simulink model "NDT_Localization"  (R2022a)
settings: Solver=FixedStepAuto  StartTime=0.0  StopTime=10.0  RelTol=1e-3
model workspace (MAT data in the model file):
  SL_ROS_VariableLengthArrays_MaxSizes : object (value not decoded)
undefined symbols (not defined in the file or in its folder): null
libraries: ros2lib x9, robotlib x8, simulink x1
(part 5 of 12)

== system NDT_Localization/observation_callback/check_localizer/If Action Subsystem/register_measurement_impl/If Action Subsystem/If Action Subsystem/solve/If Action Subsystem1/For Iterator Subsystem/compute_next_step/If Action Subsystem1/psi_t ==
  a_t : Inport
  psi : Inport  Port=2
  localizer_ptr : Inport  Port=3
  Add : Sum  Inputs=+--
  Add1 : Sum  Inputs=+-
  Bus Creator : BusCreator  Inputs=3
  Bus Selector : BusSelector  OutputSignals=phi,mu
  Bus Selector1 : BusSelector  OutputSignals=value,derivative
  Bus Selector2 : BusSelector  OutputSignals=value,derivative
  Constant : Constant  Value=0.0
  If : If  NumInputs=2  IfExpression=u1 >= u2  ShowElse=off
  Product : Product  Inputs=3
  Product1 : Product
  initial_objective_function : Subsystem
  objective_function : Subsystem  TreatAsAtomicUnit=on
  psi_t : Outport
  wires:
  psi/1 -> Bus Selector/1
  a_t/1 -> Bus Creator/1, objective_function/1(step_size), Product/2, If/1  "a_t"
  If/1 -> objective_function/Action
  Constant/1 -> initial_objective_function/1(step_size), If/2
  Bus Selector/1 -> initial_objective_function/2(phi), objective_function/2(phi)  "<phi>"
  localizer_ptr/1 -> initial_objective_function/3(localizer_ptr), objective_function/3(localizer_ptr)
  Product/1 -> Add/3
  Bus Selector/2 -> Product1/1, Product/1  "<mu>"
  objective_function/1(objective_function_value) -> Bus Selector1/1
  Bus Selector1/1 -> Add/1  "<value>"
  initial_objective_function/1(initial_objective_function_value) -> Bus Selector2/1
  Bus Selector2/1 -> Add/2  "<value>"
  Bus Selector2/2 -> Product1/2, Product/3  "<derivative>"
  Add/1 -> Bus Creator/2  "value"
  Bus Selector1/2 -> Add1/1  "<derivative>"
  Product1/1 -> Add1/2
  Add1/1 -> Bus Creator/3  "derivative"
  Bus Creator/1 -> psi_t/1

== system NDT_Localization/observation_callback/check_localizer/If Action Subsystem/register_measurement_impl/If Action Subsystem/If Action Subsystem/solve/If Action Subsystem1/For Iterator Subsystem/compute_next_step/If Action Subsystem1/For Iterator Subsystem/If Action Subsystem ==
  localizer_ptr : Inport
  phi_t : Inport  Port=2
  psi_t : Inport  Port=3
  phi : Inport  Port=4
  psi : Inport  Port=5
  f_l : Inport  Port=6
  f_u : Inport  Port=7
  aux_function : Inport  Port=8
  Action Port : ActionPort  ActionPortLabel=if(u1 > 0)
  Bus Selector : BusSelector  OutputSignals=OptimizerT.MoreThuenteLineSearch.min_step
  Data Type Conversion : DataTypeConversion  SaturateOnIntegerOverflow=off  RndMeth=Floor
  Data Type Conversion1 : DataTypeConversion  OutDataTypeStr=uint8  SaturateOnIntegerOverflow=off  RndMeth=Floor
  If : If
  If Action Subsystem : Subsystem  TreatAsAtomicUnit=on
  If Action Subsystem1 : Subsystem  TreatAsAtomicUnit=on
  If Action Subsystem2 : Subsystem  TreatAsAtomicUnit=on
  If Action Subsystem3 : Subsystem  TreatAsAtomicUnit=on
  If1 : If
  Logical Operator : Logic  Operator=OR  AllPortsSameDT=off  OutDataTypeStr=boolean
  MATLAB Function : MATLAB Function  TreatAsAtomicUnit=on
  Merge : Merge
  Relational Operator : RelationalOperator  Operator=<  OutDataTypeStr=boolean  RndMeth=Simplest  InputSameDT=off
  Out1 : Outport
  aux_function_out : Outport  Port=2
  flag : Outport  Port=3
  wires:
  localizer_ptr/1 -> If Action Subsystem3/2(localizer_ptr), Bus Selector/1
  Bus Selector/1 -> Relational Operator/2  "<min_step>"
  aux_function/1 -> If Action Subsystem3/3(aux_function), Data Type Conversion/1
  Data Type Conversion/1 -> If/1
  If/1 -> If Action Subsystem/Action
  If/2 -> If Action Subsystem1/Action
  psi_t/1 -> If Action Subsystem/1(psi_t)
  phi_t/1 -> If Action Subsystem1/1(phi_t)
  f_l/1 -> If Action Subsystem/2(f_l), If Action Subsystem1/2(f_l)
  f_u/1 -> If Action Subsystem/3(f_u), If Action Subsystem1/3(f_u)
  If Action Subsystem/1(a_t) -> Merge/1
  If Action Subsystem1/1(a_t) -> Merge/2
  Merge/1 -> Relational Operator/1, If Action Subsystem3/1(a_t), MATLAB Function/1(a_t)
  MATLAB Function/1(y) -> Logical Operator/2
  Relational Operator/1 -> Logical Operator/1
  Logical Operator/1 -> Data Type Conversion1/1
  Data Type Conversion1/1 -> If1/1
  If1/1 -> If Action Subsystem2/Action
  If1/2 -> If Action Subsystem3/Action
  If Action Subsystem2/1(a_t_out) -> flag/1
  phi/1 -> If Action Subsystem3/4(phi)
  psi/1 -> If Action Subsystem3/5(psi)

== system NDT_Localization/observation_callback/check_localizer/If Action Subsystem/register_measurement_impl/If Action Subsystem/If Action Subsystem/solve/If Action Subsystem1/For Iterator Subsystem/compute_next_step/If Action Subsystem1/f_l/initial_objective_function ==
  step_size : Inport
  phi : Inport  Port=2
  localizer_ptr : Inport  Port=3
  Add : Sum
  Add4 : Sum  Inputs=+
  Bus Creator : BusCreator  Inputs=3
  Bus Selector : BusSelector  OutputSignals=eig_pose,opt_direction,problem
  Bus Selector1 : BusSelector  OutputSignals=scan,map
  Bus Selector2 : BusSelector  OutputSignals=vx.centroid,vx.inv_covariance
  Bus Selector3 : BusSelector  OutputSignals=outlier_ratio,localizer_config.map_config.voxel_size.x,localizer_config.map_config.voxel_size.y,localizer_config.map_config.voxel_size.z
  For Iterator Subsystem : Subsystem  TreatAsAtomicUnit=on
  Math Function2 : Math  Operator=square
  Product : Product
  Product{1..9} (9 alike) : Product  Multiplication=Matrix(*)
  angle_params : Subsystem
  gradient_angle : Subsystem
  point_gradient : MATLAB Function  TreatAsAtomicUnit=on
  set_jacobian : MATLAB Function  TreatAsAtomicUnit=on
  initial_objective_function_value : Outport
  wires:
  angle_params/1(params) -> gradient_angle/1(params)
  Bus Selector3/1 -> For Iterator Subsystem/4(outlier_ratio)  "<outlier_ratio>"
  gradient_angle/3(ga_c_out) -> Product4/2
  gradient_angle/4(ga_d_out) -> Product5/2
  gradient_angle/1(ga_a_out) -> Product2/2
  gradient_angle/6(ga_f_out) -> Product7/2
  Bus Selector2/2 -> For Iterator Subsystem/3(sigma)  "<inv_covariance>"
  Product5/1 -> point_gradient/4(ga_d)
  Product3/1 -> point_gradient/2(ga_b)
  set_jacobian/1(jacobian) -> For Iterator Subsystem/8(set_jacobian)
  Bus Selector1/1 -> Product9/1, Product8/1, Product7/1, Product6/1, Product5/1, Product4/1, Product3/1, Product2/1, For Iterator Subsystem/1(data)  "<scan>"
  Bus Selector/1 -> Add/1  "<eig_pose>"
  gradient_angle/7(ga_g_out) -> Product8/2
  Product8/1 -> point_gradient/7(ga_g)
  gradient_angle/8(ga_h_out) -> Product9/2
  Math Function2/1 -> Add4/1
  Product6/1 -> point_gradient/5(ga_e)
  Bus Selector2/1 -> For Iterator Subsystem/2(myu)  "<centroid>"
  localizer_ptr/1 -> Bus Selector3/1
  gradient_angle/5(ga_e_out) -> Product6/2
  gradient_angle/2(ga_b_out) -> Product3/2
  Add/1 -> Product/1
  Bus Selector/3 -> Bus Selector1/1  "<problem>"
  Product7/1 -> point_gradient/6(ga_f)
  Product9/1 -> point_gradient/8(ga_h)
  For Iterator Subsystem/2(jacobian_out) -> Product1/1
  Product/1 -> angle_params/1(pose)  "current_state"
  Add4/1 -> Product1/2, Product/2  "step_direction"
  Product2/1 -> point_gradient/1(ga_a)
  Bus Selector/2 -> Math Function2/1  "<opt_direction>"
  Bus Creator/1 -> initial_objective_function_value/1
  Bus Selector1/2 -> Bus Selector2/1  "<map>"
  point_gradient/1(hessian) -> For Iterator Subsystem/9(set_gradient)
  Bus Selector3/3 -> For Iterator Subsystem/6(voxel_size_y)  "<y>"
  Bus Selector3/4 -> For Iterator Subsystem/7(voxel_size_z)  "<z>"
  phi/1 -> Bus Selector/1
  Bus Selector3/2 -> For Iterator Subsystem/5(voxel_size_x)  "<x>"
  Product4/1 -> point_gradient/3(ga_c)
  step_size/1 -> Bus Creator/1, Add/2  "step_size"
  For Iterator Subsystem/1(score_out) -> Bus Creator/2  "value"
  Product1/1 -> Bus Creator/3  "derivative"

== system NDT_Localization/observation_callback/check_localizer/If Action Subsystem/register_measurement_impl/If Action Subsystem/If Action Subsystem/solve/If Action Subsystem1/For Iterator Subsystem/compute_next_step/If Action Subsystem1/f_l/objective_function ==
  step_size : Inport
  phi : Inport  Port=2
  localizer_ptr : Inport  Port=3
  Action Port : ActionPort
  Add : Sum
  Add4 : Sum  Inputs=+
  Bus Creator : BusCreator  Inputs=3
  Bus Selector : BusSelector  OutputSignals=eig_pose,opt_direction,problem
  Bus Selector1 : BusSelector  OutputSignals=scan,map
  Bus Selector2 : BusSelector  OutputSignals=vx.centroid,vx.inv_covariance
  Bus Selector3 : BusSelector  OutputSignals=outlier_ratio,localizer_config.map_config.voxel_size.x,localizer_config.map_config.voxel_size.y,localizer_config.map_config.voxel_size.z
  For Iterator Subsystem : Subsystem  TreatAsAtomicUnit=on
  Math Function2 : Math  Operator=square
  Product : Product
  Product{1..9} (9 alike) : Product  Multiplication=Matrix(*)
  angle_params : Subsystem
  gradient_angle : Subsystem
  point_gradient : MATLAB Function  TreatAsAtomicUnit=on
  set_jacobian : MATLAB Function  TreatAsAtomicUnit=on
  objective_function_value : Outport
  wires:
  Add/1 -> Product/1
  step_size/1 -> Bus Creator/1, Add/2  "step_size"
  Product/1 -> angle_params/1(pose)  "current_state"
  Bus Selector/1 -> Add/1  "<eig_pose>"
  Add4/1 -> Product1/2, Product/2  "step_direction"
  phi/1 -> Bus Selector/1
  Bus Selector/2 -> Math Function2/1  "<opt_direction>"
  Math Function2/1 -> Add4/1
  Bus Selector/3 -> Bus Selector1/1  "<problem>"
  For Iterator Subsystem/2(jacobian_out) -> Product1/1
  Product1/1 -> Bus Creator/3  "derivative"
  Product9/1 -> point_gradient/8(ga_h)
  Product8/1 -> point_gradient/7(ga_g)
  Bus Selector2/2 -> For Iterator Subsystem/3(sigma)  "<inv_covariance>"
  gradient_angle/4(ga_d_out) -> Product5/2
  Product7/1 -> point_gradient/6(ga_f)
  Product6/1 -> point_gradient/5(ga_e)
  gradient_angle/6(ga_f_out) -> Product7/2
  Bus Selector1/1 -> Product9/1, Product8/1, Product7/1, Product6/1, Product5/1, Product4/1, Product3/1, Product2/1, For Iterator Subsystem/1(data)  "<scan>"
  point_gradient/1(hessian) -> For Iterator Subsystem/9(set_gradient)
  gradient_angle/2(ga_b_out) -> Product3/2
  gradient_angle/3(ga_c_out) -> Product4/2
  gradient_angle/7(ga_g_out) -> Product8/2
  gradient_angle/5(ga_e_out) -> Product6/2
  gradient_angle/8(ga_h_out) -> Product9/2
  Product5/1 -> point_gradient/4(ga_d)
  Product3/1 -> point_gradient/2(ga_b)
  Product4/1 -> point_gradient/3(ga_c)
  angle_params/1(params) -> gradient_angle/1(params)
  set_jacobian/1(jacobian) -> For Iterator Subsystem/8(set_jacobian)
  Bus Selector1/2 -> Bus Selector2/1  "<map>"
  gradient_angle/1(ga_a_out) -> Product2/2
  Product2/1 -> point_gradient/1(ga_a)
  Bus Selector2/1 -> For Iterator Subsystem/2(myu)  "<centroid>"
  localizer_ptr/1 -> Bus Selector3/1
  Bus Selector3/1 -> For Iterator Subsystem/4(outlier_ratio)  "<outlier_ratio>"
  Bus Selector3/2 -> For Iterator Subsystem/5(voxel_size_x)  "<x>"
  Bus Selector3/3 -> For Iterator Subsystem/6(voxel_size_y)  "<y>"
  Bus Selector3/4 -> For Iterator Subsystem/7(voxel_size_z)  "<z>"
  For Iterator Subsystem/1(score_out) -> Bus Creator/2  "value"
  Bus Creator/1 -> objective_function_value/1

== system NDT_Localization/observation_callback/check_localizer/If Action Subsystem/register_measurement_impl/If Action Subsystem/If Action Subsystem/solve/If Action Subsystem1/For Iterator Subsystem/compute_next_step/If Action Subsystem1/f_u/initial_objective_function ==
  step_size : Inport
  phi : Inport  Port=2
  localizer_ptr : Inport  Port=3
  Add : Sum
  Add4 : Sum  Inputs=+
  Bus Creator : BusCreator  Inputs=3
  Bus Selector : BusSelector  OutputSignals=eig_pose,opt_direction,problem
  Bus Selector1 : BusSelector  OutputSignals=scan,map
  Bus Selector2 : BusSelector  OutputSignals=vx.centroid,vx.inv_covariance
  Bus Selector3 : BusSelector  OutputSignals=outlier_ratio,localizer_config.map_config.voxel_size.x,localizer_config.map_config.voxel_size.y,localizer_config.map_config.voxel_size.z
  For Iterator Subsystem : Subsystem  TreatAsAtomicUnit=on
  Math Function2 : Math  Operator=square
  Product : Product
  Product{1..9} (9 alike) : Product  Multiplication=Matrix(*)
  angle_params : Subsystem
  gradient_angle : Subsystem
  point_gradient : MATLAB Function  TreatAsAtomicUnit=on
  set_jacobian : MATLAB Function  TreatAsAtomicUnit=on
  initial_objective_function_value : Outport
  wires:
  angle_params/1(params) -> gradient_angle/1(params)
  Bus Selector3/1 -> For Iterator Subsystem/4(outlier_ratio)  "<outlier_ratio>"
  gradient_angle/3(ga_c_out) -> Product4/2
  gradient_angle/4(ga_d_out) -> Product5/2
  gradient_angle/1(ga_a_out) -> Product2/2
  gradient_angle/6(ga_f_out) -> Product7/2
  Bus Selector2/2 -> For Iterator Subsystem/3(sigma)  "<inv_covariance>"
  Product5/1 -> point_gradient/4(ga_d)
  Product3/1 -> point_gradient/2(ga_b)
  set_jacobian/1(jacobian) -> For Iterator Subsystem/8(set_jacobian)
  Bus Selector1/1 -> Product9/1, Product8/1, Product7/1, Product6/1, Product5/1, Product4/1, Product3/1, Product2/1, For Iterator Subsystem/1(data)  "<scan>"
  Bus Selector/1 -> Add/1  "<eig_pose>"
  gradient_angle/7(ga_g_out) -> Product8/2
  Product8/1 -> point_gradient/7(ga_g)
  gradient_angle/8(ga_h_out) -> Product9/2
  Math Function2/1 -> Add4/1
  Product6/1 -> point_gradient/5(ga_e)
  Bus Selector2/1 -> For Iterator Subsystem/2(myu)  "<centroid>"
  localizer_ptr/1 -> Bus Selector3/1
  gradient_angle/5(ga_e_out) -> Product6/2
  gradient_angle/2(ga_b_out) -> Product3/2
  Add/1 -> Product/1
  Bus Selector/3 -> Bus Selector1/1  "<problem>"
  Product7/1 -> point_gradient/6(ga_f)
  Product9/1 -> point_gradient/8(ga_h)
  For Iterator Subsystem/2(jacobian_out) -> Product1/1
  Product/1 -> angle_params/1(pose)  "current_state"
  Add4/1 -> Product1/2, Product/2  "step_direction"
  Product2/1 -> point_gradient/1(ga_a)
  Bus Selector/2 -> Math Function2/1  "<opt_direction>"
  Bus Creator/1 -> initial_objective_function_value/1
  Bus Selector1/2 -> Bus Selector2/1  "<map>"
  point_gradient/1(hessian) -> For Iterator Subsystem/9(set_gradient)
  Bus Selector3/3 -> For Iterator Subsystem/6(voxel_size_y)  "<y>"
  Bus Selector3/4 -> For Iterator Subsystem/7(voxel_size_z)  "<z>"
  phi/1 -> Bus Selector/1
  Bus Selector3/2 -> For Iterator Subsystem/5(voxel_size_x)  "<x>"
  Product4/1 -> point_gradient/3(ga_c)
  step_size/1 -> Bus Creator/1, Add/2  "step_size"
  For Iterator Subsystem/1(score_out) -> Bus Creator/2  "value"
  Product1/1 -> Bus Creator/3  "derivative"

== system NDT_Localization/observation_callback/check_localizer/If Action Subsystem/register_measurement_impl/If Action Subsystem/If Action Subsystem/solve/If Action Subsystem1/For Iterator Subsystem/compute_next_step/If Action Subsystem1/f_u/objective_function ==
  step_size : Inport
  phi : Inport  Port=2
  localizer_ptr : Inport  Port=3
  Action Port : ActionPort
  Add : Sum
  Add4 : Sum  Inputs=+
  Bus Creator : BusCreator  Inputs=3
  Bus Selector : BusSelector  OutputSignals=eig_pose,opt_direction,problem
  Bus Selector1 : BusSelector  OutputSignals=scan,map
  Bus Selector2 : BusSelector  OutputSignals=vx.centroid,vx.inv_covariance
  Bus Selector3 : BusSelector  OutputSignals=outlier_ratio,localizer_config.map_config.voxel_size.x,localizer_config.map_config.voxel_size.y,localizer_config.map_config.voxel_size.z
  For Iterator Subsystem : Subsystem  TreatAsAtomicUnit=on
  Math Function2 : Math  Operator=square
  Product : Product
  Product{1..9} (9 alike) : Product  Multiplication=Matrix(*)
  angle_params : Subsystem
  gradient_angle : Subsystem
  point_gradient : MATLAB Function  TreatAsAtomicUnit=on
  set_jacobian : MATLAB Function  TreatAsAtomicUnit=on
  objective_function_value : Outport
  wires:
  Add/1 -> Product/1
  step_size/1 -> Bus Creator/1, Add/2  "step_size"
  Product/1 -> angle_params/1(pose)  "current_state"
  Bus Selector/1 -> Add/1  "<eig_pose>"
  Add4/1 -> Product1/2, Product/2  "step_direction"
  phi/1 -> Bus Selector/1
  Bus Selector/2 -> Math Function2/1  "<opt_direction>"
  Math Function2/1 -> Add4/1
  Bus Selector/3 -> Bus Selector1/1  "<problem>"
  For Iterator Subsystem/2(jacobian_out) -> Product1/1
  Product1/1 -> Bus Creator/3  "derivative"
  Product9/1 -> point_gradient/8(ga_h)
  Product8/1 -> point_gradient/7(ga_g)
  Bus Selector2/2 -> For Iterator Subsystem/3(sigma)  "<inv_covariance>"
  gradient_angle/4(ga_d_out) -> Product5/2
  Product7/1 -> point_gradient/6(ga_f)
  Product6/1 -> point_gradient/5(ga_e)
  gradient_angle/6(ga_f_out) -> Product7/2
  Bus Selector1/1 -> Product9/1, Product8/1, Product7/1, Product6/1, Product5/1, Product4/1, Product3/1, Product2/1, For Iterator Subsystem/1(data)  "<scan>"
  point_gradient/1(hessian) -> For Iterator Subsystem/9(set_gradient)
  gradient_angle/2(ga_b_out) -> Product3/2
  gradient_angle/3(ga_c_out) -> Product4/2
  gradient_angle/7(ga_g_out) -> Product8/2
  gradient_angle/5(ga_e_out) -> Product6/2
  gradient_angle/8(ga_h_out) -> Product9/2
  Product5/1 -> point_gradient/4(ga_d)
  Product3/1 -> point_gradient/2(ga_b)
  Product4/1 -> point_gradient/3(ga_c)
  angle_params/1(params) -> gradient_angle/1(params)
  set_jacobian/1(jacobian) -> For Iterator Subsystem/8(set_jacobian)
  Bus Selector1/2 -> Bus Selector2/1  "<map>"
  gradient_angle/1(ga_a_out) -> Product2/2
  Product2/1 -> point_gradient/1(ga_a)
  Bus Selector2/1 -> For Iterator Subsystem/2(myu)  "<centroid>"
  localizer_ptr/1 -> Bus Selector3/1
  Bus Selector3/1 -> For Iterator Subsystem/4(outlier_ratio)  "<outlier_ratio>"
  Bus Selector3/2 -> For Iterator Subsystem/5(voxel_size_x)  "<x>"
  Bus Selector3/3 -> For Iterator Subsystem/6(voxel_size_y)  "<y>"
  Bus Selector3/4 -> For Iterator Subsystem/7(voxel_size_z)  "<z>"
  For Iterator Subsystem/1(score_out) -> Bus Creator/2  "value"
  Bus Creator/1 -> objective_function_value/1

== system NDT_Localization/observation_callback/check_localizer/If Action Subsystem/register_measurement_impl/If Action Subsystem/If Action Subsystem/solve/If Action Subsystem1/For Iterator Subsystem/compute_next_step/If Action Subsystem1/phi_0/For Iterator Subsystem ==
  data : Inport
  myu : Inport  Port=2
  sigma : Inport  Port=3
  outlier_ratio : Inport  Port=4
  voxel_size_x : Inport  Port=5
  voxel_size_y : Inport  Port=6
  voxel_size_z : Inport  Port=7
  set_jacobian : Inport  Port=8
  set_gradient : Inport  Port=9
  Affine : MATLAB Function  TreatAsAtomicUnit=on
  Delay : Delay  DelayLength=1
  For Iterator : ForIterator  IterationSource=external
  MATLAB Function : MATLAB Function  TreatAsAtomicUnit=on
  Width : Width
  gradient_jaco : Subsystem
  make_c_param : Subsystem
  make_d_param : Subsystem
  score : Subsystem
  score_out : Outport
  jacobian_out : Outport  Port=2
  wires:
  make_c_param/1(c1) -> make_d_param/1(c1)
  voxel_size_z/1 -> make_c_param/4(voxel_size_z)
  outlier_ratio/1 -> make_c_param/1(outlier_ratio)
  make_d_param/2(d2) -> gradient_jaco/9(d2), score/6(d2)
  voxel_size_y/1 -> make_c_param/3(voxel_size_y)
  make_c_param/2(c2) -> make_d_param/2(c2)
  voxel_size_x/1 -> make_c_param/2(voxel_size_x)
  make_d_param/1(d1) -> score/5(d1), gradient_jaco/8(d1)
  Width/1 -> For Iterator/1
  For Iterator/1 -> gradient_jaco/3(index), MATLAB Function/2(index)
  MATLAB Function/1(pt) -> Affine/1(u)
  Affine/1(out) -> score/4(x), gradient_jaco/4(data)
  sigma/1 -> score/2(sigma), gradient_jaco/5(sigma)
  myu/1 -> gradient_jaco/6(myu), score/3(myu)
  score/1(p) -> score_out/1, Delay/1
  Delay/1 -> score/1(score)
  set_jacobian/1 -> gradient_jaco/1(set_jacobian)
  gradient_jaco/1(Out1) -> jacobian_out/1
  set_gradient/1 -> gradient_jaco/2(set_gradient)
  data/1 -> gradient_jaco/7(x), MATLAB Function/1(data), Width/1

== system NDT_Localization/observation_callback/check_localizer/If Action Subsystem/register_measurement_impl/If Action Subsystem/If Action Subsystem/solve/If Action Subsystem1/For Iterator Subsystem/compute_next_step/If Action Subsystem1/phi_0/angle_params ==
  pose : Inport
  Bus Creator : BusCreator  Inputs=6
  If : If  NumInputs=2  IfExpression=u1 > u2
  If Action Subsystem : Subsystem  TreatAsAtomicUnit=on
  If Action Subsystem1 : Subsystem  TreatAsAtomicUnit=on
  If Action Subsystem2 : Subsystem  TreatAsAtomicUnit=on
  If Action Subsystem3 : Subsystem  TreatAsAtomicUnit=on
  If Action Subsystem4 : Subsystem  TreatAsAtomicUnit=on
  If Action Subsystem5 : Subsystem  TreatAsAtomicUnit=on
  If1 : If  NumInputs=2  IfExpression=u1 > u2
  If2 : If  NumInputs=2  IfExpression=u1 > u2
  MATLAB Function : MATLAB Function  TreatAsAtomicUnit=on
  Merge{,1..5} (6 alike) : Merge
  approx_thresh : Constant  Value=0.00010
  params : Outport
  wires:
  pose/1 -> MATLAB Function/1(u)
  MATLAB Function/1(x) -> If/2, If Action Subsystem1/1(x)
  MATLAB Function/3(z) -> If2/2, If Action Subsystem5/1(z)
  MATLAB Function/2(y) -> If Action Subsystem3/1(y), If1/2
  If Action Subsystem1/1(Out1) -> Merge/2
  If Action Subsystem1/2(Out2) -> Merge1/2
  If Action Subsystem3/1(Out1) -> Merge2/2
  If Action Subsystem3/2(Out2) -> Merge3/2
  If Action Subsystem5/1(Out1) -> Merge4/2
  If Action Subsystem5/2(Out2) -> Merge5/2
  approx_thresh/1 -> If2/1, If1/1, If/1
  If/1 -> If Action Subsystem/Action
  If/2 -> If Action Subsystem1/Action
  If1/1 -> If Action Subsystem2/Action
  If1/2 -> If Action Subsystem3/Action
  If2/2 -> If Action Subsystem5/Action
  If2/1 -> If Action Subsystem4/Action
  If Action Subsystem/1(Out1) -> Merge/1
  If Action Subsystem/2(Out2) -> Merge1/1
  If Action Subsystem2/1(Out1) -> Merge2/1
  If Action Subsystem2/2(Out2) -> Merge3/1
  If Action Subsystem4/1(Out1) -> Merge4/1
  If Action Subsystem4/2(Out2) -> Merge5/1
  Bus Creator/1 -> params/1
  Merge/1 -> Bus Creator/1  "cx"
  Merge1/1 -> Bus Creator/2  "sx"
  Merge2/1 -> Bus Creator/3  "cy"
  Merge3/1 -> Bus Creator/4  "sy"
  Merge4/1 -> Bus Creator/5  "cz"
  Merge5/1 -> Bus Creator/6  "sz"

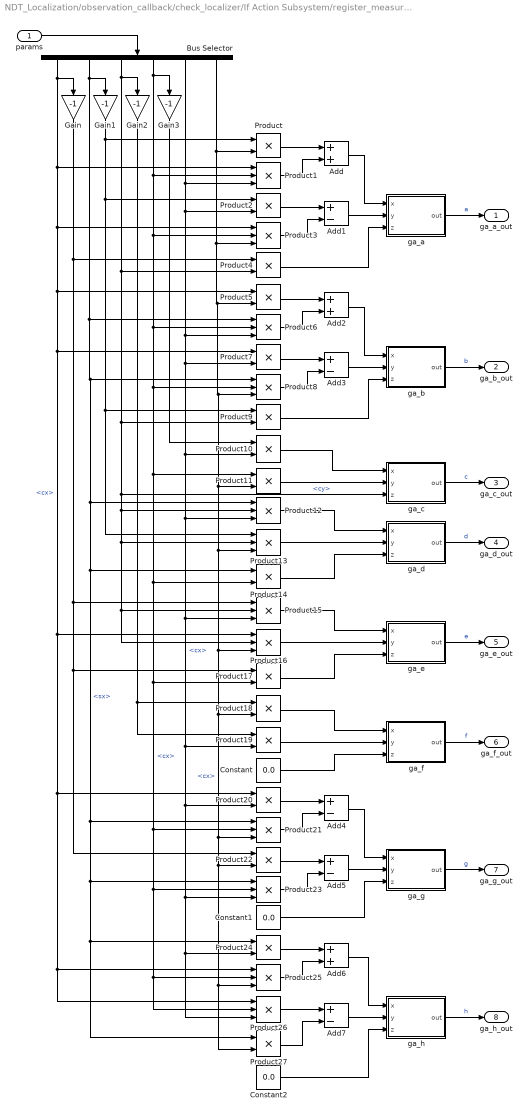
== system NDT_Localization/observation_callback/check_localizer/If Action Subsystem/register_measurement_impl/If Action Subsystem/If Action Subsystem/solve/If Action Subsystem1/For Iterator Subsystem/compute_next_step/If Action Subsystem1/phi_0/gradient_angle ==
  params : Inport
  Add : Sum
  Add{1,3..5,7} (5 alike) : Sum  Inputs=+-
  Add2 : Sum
  Add6 : Sum
  Bus Selector : BusSelector  OutputSignals=cx,sx,cy,sy,cz,sz
  Constant : Constant  Value=0.0
  Constant1 : Constant  Value=0.0
  Constant2 : Constant  Value=0.0
  Gain{,1..3} (4 alike) : Gain  Gain=-1
  Product{,2,4..5,7,9..11,14,17..20,22,24,27} (16 alike) : Product
  Product{1,3,6,8,12..13,15..16,21,23,25..26} (12 alike) : Product  Inputs=3
  ga_a : MATLAB Function  TreatAsAtomicUnit=on
  ga_b : MATLAB Function  TreatAsAtomicUnit=on
  ga_c : MATLAB Function  TreatAsAtomicUnit=on
  ga_d : MATLAB Function  TreatAsAtomicUnit=on
  ga_e : MATLAB Function  TreatAsAtomicUnit=on
  ga_f : MATLAB Function  TreatAsAtomicUnit=on
  ga_g : MATLAB Function  TreatAsAtomicUnit=on
  ga_h : MATLAB Function  TreatAsAtomicUnit=on
  ga_a_out : Outport
  ga_b_out : Outport  Port=2
  ga_c_out : Outport  Port=3
  ga_d_out : Outport  Port=4
  ga_e_out : Outport  Port=5
  ga_f_out : Outport  Port=6
  ga_g_out : Outport  Port=7
  ga_h_out : Outport  Port=8
  wires:
  params/1 -> Bus Selector/1
  Bus Selector/1 -> Product1/1, Product16/1, Product25/1, Product26/1, Product20/1, Product7/1, Product5/1, Product3/1, Gain/1  "<cx>"
  Bus Selector/2 -> Product6/1, Product12/1, Product14/1, Product21/1, Product23/1, Product27/1, Product24/1, Product8/1, Gain1/1  "<sx>"
  Bus Selector/3 -> Product12/2, Product13/2, Product15/2, Product16/2, ga_c/3(z), Product9/2, Product4/2, Gain2/1  "<cy>"
  Bus Selector/4 -> Product11/1, Product14/2, Product17/2, Product21/2, Product25/2, Product26/2, Product23/2, Product8/2, Product6/2, Product3/2, Product1/2, Gain3/1  "<cx>"
  Bus Selector/5 -> Product6/3, Product10/2, Product12/3, Product15/3, Product19/2, Product20/2, Product23/3, Product26/3, Product24/2, Product7/2, Product2/2, Product1/3  "<cx>"
  Bus Selector/6 -> Product11/2, Product13/3, Product16/3, Product18/2, Product21/3, Product22/2, Product25/3, Product27/2, Product8/3, Product5/2, Product3/3, Product/2  "<cx>"
  Gain1/1 -> Product13/1, Product9/1, Product2/1, Product/1
  Product/1 -> Add/1
  Product1/1 -> Add/2
  Product2/1 -> Add1/1
  Add/1 -> ga_a/1(x)
  Add1/1 -> ga_a/2(y)
  Gain/1 -> Product15/1, Product17/1, Product22/1, Product4/1
  Product4/1 -> ga_a/3(z)
  Product3/1 -> Add1/2
  Product6/1 -> Add2/2
  Product7/1 -> Add3/1
  Product8/1 -> Add3/2
  Product5/1 -> Add2/1
  Add2/1 -> ga_b/1(x)
  Product9/1 -> ga_b/3(z)
  Add3/1 -> ga_b/2(y)
  Product11/1 -> ga_c/2(y)
  Product10/1 -> ga_c/1(x)
  Gain2/1 -> Product18/1, Product19/1
  Gain3/1 -> Product10/1
  Product13/1 -> ga_d/2(y)
  Product12/1 -> ga_d/1(x)
  Product14/1 -> ga_d/3(z)
  Product19/1 -> ga_f/2(y)
  Constant/1 -> ga_f/3(z)
  Product18/1 -> ga_f/1(x)
  Product16/1 -> ga_e/2(y)
  Product17/1 -> ga_e/3(z)
  Product15/1 -> ga_e/1(x)
  Product21/1 -> Add4/2
  Product22/1 -> Add5/1
  Product23/1 -> Add5/2
  Product20/1 -> Add4/1
  Add5/1 -> ga_g/2(y)
  Product25/1 -> Add6/2
  Product26/1 -> Add7/1
  Product27/1 -> Add7/2
  Product24/1 -> Add6/1
  Constant1/1 -> ga_g/3(z)
  Add4/1 -> ga_g/1(x)
  Add7/1 -> ga_h/2(y)
  Add6/1 -> ga_h/1(x)
  Constant2/1 -> ga_h/3(z)
  ga_a/1(out) -> ga_a_out/1  "a"
  ga_b/1(out) -> ga_b_out/1  "b"
  ga_c/1(out) -> ga_c_out/1  "c"
  ga_d/1(out) -> ga_d_out/1  "d"
  ga_e/1(out) -> ga_e_out/1  "e"
  ga_f/1(out) -> ga_f_out/1  "f"
  ga_g/1(out) -> ga_g_out/1  "g"
  ga_h/1(out) -> ga_h_out/1  "h"

== system NDT_Localization/observation_callback/check_localizer/If Action Subsystem/register_measurement_impl/If Action Subsystem/If Action Subsystem/solve/If Action Subsystem1/For Iterator Subsystem/compute_next_step/If Action Subsystem1/phi_t/For Iterator Subsystem ==
  data : Inport
  myu : Inport  Port=2
  sigma : Inport  Port=3
  outlier_ratio : Inport  Port=4
  voxel_size_x : Inport  Port=5
  voxel_size_y : Inport  Port=6
  voxel_size_z : Inport  Port=7
  set_jacobian : Inport  Port=8
  set_gradient : Inport  Port=9
  Affine : MATLAB Function  TreatAsAtomicUnit=on
  Delay : Delay  DelayLength=1
  For Iterator : ForIterator  IterationSource=external
  MATLAB Function : MATLAB Function  TreatAsAtomicUnit=on
  Width : Width
  gradient_jaco : Subsystem
  make_c_param : Subsystem
  make_d_param : Subsystem
  score : Subsystem
  score_out : Outport
  jacobian_out : Outport  Port=2
  wires:
  make_c_param/1(c1) -> make_d_param/1(c1)
  voxel_size_z/1 -> make_c_param/4(voxel_size_z)
  outlier_ratio/1 -> make_c_param/1(outlier_ratio)
  make_d_param/2(d2) -> gradient_jaco/9(d2), score/6(d2)
  voxel_size_y/1 -> make_c_param/3(voxel_size_y)
  make_c_param/2(c2) -> make_d_param/2(c2)
  voxel_size_x/1 -> make_c_param/2(voxel_size_x)
  make_d_param/1(d1) -> score/5(d1), gradient_jaco/8(d1)
  Width/1 -> For Iterator/1
  For Iterator/1 -> gradient_jaco/3(index), MATLAB Function/2(index)
  MATLAB Function/1(pt) -> Affine/1(u)
  Affine/1(out) -> score/4(x), gradient_jaco/4(data)
  sigma/1 -> score/2(sigma), gradient_jaco/5(sigma)
  myu/1 -> gradient_jaco/6(myu), score/3(myu)
  score/1(p) -> score_out/1, Delay/1
  Delay/1 -> score/1(score)
  set_jacobian/1 -> gradient_jaco/1(set_jacobian)
  gradient_jaco/1(Out1) -> jacobian_out/1
  set_gradient/1 -> gradient_jaco/2(set_gradient)
  data/1 -> gradient_jaco/7(x), MATLAB Function/1(data), Width/1

== system NDT_Localization/observation_callback/check_localizer/If Action Subsystem/register_measurement_impl/If Action Subsystem/If Action Subsystem/solve/If Action Subsystem1/For Iterator Subsystem/compute_next_step/If Action Subsystem1/phi_t/angle_params ==
  pose : Inport
  Bus Creator : BusCreator  Inputs=6
  If : If  NumInputs=2  IfExpression=u1 > u2
  If Action Subsystem : Subsystem  TreatAsAtomicUnit=on
  If Action Subsystem1 : Subsystem  TreatAsAtomicUnit=on
  If Action Subsystem2 : Subsystem  TreatAsAtomicUnit=on
  If Action Subsystem3 : Subsystem  TreatAsAtomicUnit=on
  If Action Subsystem4 : Subsystem  TreatAsAtomicUnit=on
  If Action Subsystem5 : Subsystem  TreatAsAtomicUnit=on
  If1 : If  NumInputs=2  IfExpression=u1 > u2
  If2 : If  NumInputs=2  IfExpression=u1 > u2
  MATLAB Function : MATLAB Function  TreatAsAtomicUnit=on
  Merge{,1..5} (6 alike) : Merge
  approx_thresh : Constant  Value=0.00010
  params : Outport
  wires:
  pose/1 -> MATLAB Function/1(u)
  MATLAB Function/1(x) -> If/2, If Action Subsystem1/1(x)
  MATLAB Function/3(z) -> If2/2, If Action Subsystem5/1(z)
  MATLAB Function/2(y) -> If Action Subsystem3/1(y), If1/2
  If Action Subsystem1/1(Out1) -> Merge/2
  If Action Subsystem1/2(Out2) -> Merge1/2
  If Action Subsystem3/1(Out1) -> Merge2/2
  If Action Subsystem3/2(Out2) -> Merge3/2
  If Action Subsystem5/1(Out1) -> Merge4/2
  If Action Subsystem5/2(Out2) -> Merge5/2
  approx_thresh/1 -> If2/1, If1/1, If/1
  If/1 -> If Action Subsystem/Action
  If/2 -> If Action Subsystem1/Action
  If1/1 -> If Action Subsystem2/Action
  If1/2 -> If Action Subsystem3/Action
  If2/2 -> If Action Subsystem5/Action
  If2/1 -> If Action Subsystem4/Action
  If Action Subsystem/1(Out1) -> Merge/1
  If Action Subsystem/2(Out2) -> Merge1/1
  If Action Subsystem2/1(Out1) -> Merge2/1
  If Action Subsystem2/2(Out2) -> Merge3/1
  If Action Subsystem4/1(Out1) -> Merge4/1
  If Action Subsystem4/2(Out2) -> Merge5/1
  Bus Creator/1 -> params/1
  Merge/1 -> Bus Creator/1  "cx"
  Merge1/1 -> Bus Creator/2  "sx"
  Merge2/1 -> Bus Creator/3  "cy"
  Merge3/1 -> Bus Creator/4  "sy"
  Merge4/1 -> Bus Creator/5  "cz"
  Merge5/1 -> Bus Creator/6  "sz"

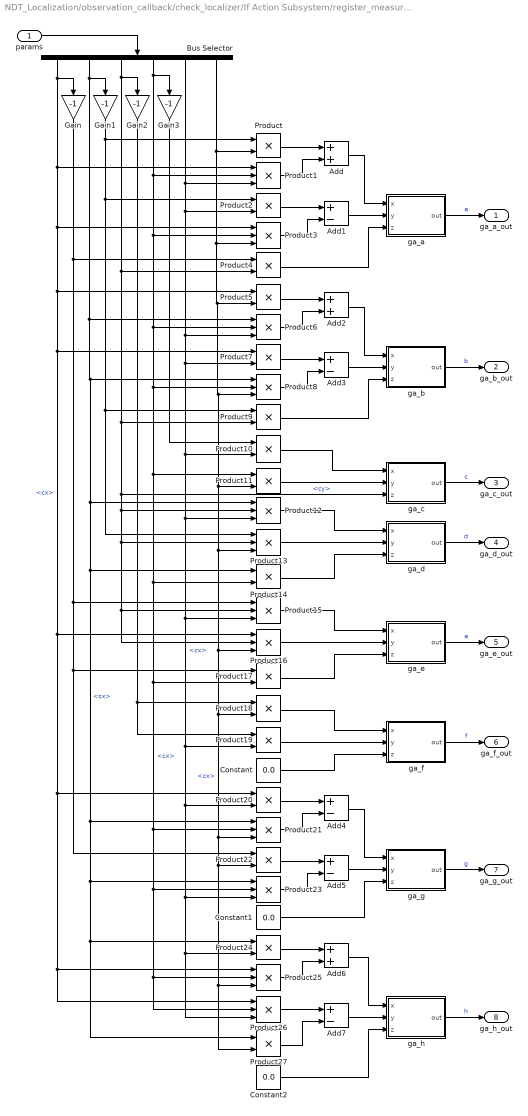
== system NDT_Localization/observation_callback/check_localizer/If Action Subsystem/register_measurement_impl/If Action Subsystem/If Action Subsystem/solve/If Action Subsystem1/For Iterator Subsystem/compute_next_step/If Action Subsystem1/phi_t/gradient_angle ==
  params : Inport
  Add : Sum
  Add{1,3..5,7} (5 alike) : Sum  Inputs=+-
  Add2 : Sum
  Add6 : Sum
  Bus Selector : BusSelector  OutputSignals=cx,sx,cy,sy,cz,sz
  Constant : Constant  Value=0.0
  Constant1 : Constant  Value=0.0
  Constant2 : Constant  Value=0.0
  Gain{,1..3} (4 alike) : Gain  Gain=-1
  Product{,2,4..5,7,9..11,14,17..20,22,24,27} (16 alike) : Product
  Product{1,3,6,8,12..13,15..16,21,23,25..26} (12 alike) : Product  Inputs=3
  ga_a : MATLAB Function  TreatAsAtomicUnit=on
  ga_b : MATLAB Function  TreatAsAtomicUnit=on
  ga_c : MATLAB Function  TreatAsAtomicUnit=on
  ga_d : MATLAB Function  TreatAsAtomicUnit=on
  ga_e : MATLAB Function  TreatAsAtomicUnit=on
  ga_f : MATLAB Function  TreatAsAtomicUnit=on
  ga_g : MATLAB Function  TreatAsAtomicUnit=on
  ga_h : MATLAB Function  TreatAsAtomicUnit=on
  ga_a_out : Outport
  ga_b_out : Outport  Port=2
  ga_c_out : Outport  Port=3
  ga_d_out : Outport  Port=4
  ga_e_out : Outport  Port=5
  ga_f_out : Outport  Port=6
  ga_g_out : Outport  Port=7
  ga_h_out : Outport  Port=8
  wires:
  params/1 -> Bus Selector/1
  Bus Selector/1 -> Product1/1, Product16/1, Product25/1, Product26/1, Product20/1, Product7/1, Product5/1, Product3/1, Gain/1  "<cx>"
  Bus Selector/2 -> Product6/1, Product12/1, Product14/1, Product21/1, Product23/1, Product27/1, Product24/1, Product8/1, Gain1/1  "<sx>"
  Bus Selector/3 -> Product12/2, Product13/2, Product15/2, Product16/2, ga_c/3(z), Product9/2, Product4/2, Gain2/1  "<cy>"
  Bus Selector/4 -> Product11/1, Product14/2, Product17/2, Product21/2, Product25/2, Product26/2, Product23/2, Product8/2, Product6/2, Product3/2, Product1/2, Gain3/1  "<cx>"
  Bus Selector/5 -> Product6/3, Product10/2, Product12/3, Product15/3, Product19/2, Product20/2, Product23/3, Product26/3, Product24/2, Product7/2, Product2/2, Product1/3  "<cx>"
  Bus Selector/6 -> Product11/2, Product13/3, Product16/3, Product18/2, Product21/3, Product22/2, Product25/3, Product27/2, Product8/3, Product5/2, Product3/3, Product/2  "<cx>"
  Gain1/1 -> Product13/1, Product9/1, Product2/1, Product/1
  Product/1 -> Add/1
  Product1/1 -> Add/2
  Product2/1 -> Add1/1
  Add/1 -> ga_a/1(x)
  Add1/1 -> ga_a/2(y)
  Gain/1 -> Product15/1, Product17/1, Product22/1, Product4/1
  Product4/1 -> ga_a/3(z)
  Product3/1 -> Add1/2
  Product6/1 -> Add2/2
  Product7/1 -> Add3/1
  Product8/1 -> Add3/2
  Product5/1 -> Add2/1
  Add2/1 -> ga_b/1(x)
  Product9/1 -> ga_b/3(z)
  Add3/1 -> ga_b/2(y)
  Product11/1 -> ga_c/2(y)
  Product10/1 -> ga_c/1(x)
  Gain2/1 -> Product18/1, Product19/1
  Gain3/1 -> Product10/1
  Product13/1 -> ga_d/2(y)
  Product12/1 -> ga_d/1(x)
  Product14/1 -> ga_d/3(z)
  Product19/1 -> ga_f/2(y)
  Constant/1 -> ga_f/3(z)
  Product18/1 -> ga_f/1(x)
  Product16/1 -> ga_e/2(y)
  Product17/1 -> ga_e/3(z)
  Product15/1 -> ga_e/1(x)
  Product21/1 -> Add4/2
  Product22/1 -> Add5/1
  Product23/1 -> Add5/2
  Product20/1 -> Add4/1
  Add5/1 -> ga_g/2(y)
  Product25/1 -> Add6/2
  Product26/1 -> Add7/1
  Product27/1 -> Add7/2
  Product24/1 -> Add6/1
  Constant1/1 -> ga_g/3(z)
  Add4/1 -> ga_g/1(x)
  Add7/1 -> ga_h/2(y)
  Add6/1 -> ga_h/1(x)
  Constant2/1 -> ga_h/3(z)
  ga_a/1(out) -> ga_a_out/1  "a"
  ga_b/1(out) -> ga_b_out/1  "b"
  ga_c/1(out) -> ga_c_out/1  "c"
  ga_d/1(out) -> ga_d_out/1  "d"
  ga_e/1(out) -> ga_e_out/1  "e"
  ga_f/1(out) -> ga_f_out/1  "f"
  ga_g/1(out) -> ga_g_out/1  "g"
  ga_h/1(out) -> ga_h_out/1  "h"

== system NDT_Localization/observation_callback/check_localizer/If Action Subsystem/register_measurement_impl/If Action Subsystem/If Action Subsystem/solve/If Action Subsystem1/For Iterator Subsystem/compute_next_step/If Action Subsystem1/psi_t/initial_objective_function ==
  step_size : Inport
  phi : Inport  Port=2
  localizer_ptr : Inport  Port=3
  Add : Sum
  Add4 : Sum  Inputs=+
  Bus Creator : BusCreator  Inputs=3
  Bus Selector : BusSelector  OutputSignals=eig_pose,opt_direction,problem
  Bus Selector1 : BusSelector  OutputSignals=scan,map
  Bus Selector2 : BusSelector  OutputSignals=vx.centroid,vx.inv_covariance
  Bus Selector3 : BusSelector  OutputSignals=outlier_ratio,localizer_config.map_config.voxel_size.x,localizer_config.map_config.voxel_size.y,localizer_config.map_config.voxel_size.z
  For Iterator Subsystem : Subsystem  TreatAsAtomicUnit=on
  Math Function2 : Math  Operator=square
  Product : Product
  Product{1..9} (9 alike) : Product  Multiplication=Matrix(*)
  angle_params : Subsystem
  gradient_angle : Subsystem
  point_gradient : MATLAB Function  TreatAsAtomicUnit=on
  set_jacobian : MATLAB Function  TreatAsAtomicUnit=on
  initial_objective_function_value : Outport
  wires:
  angle_params/1(params) -> gradient_angle/1(params)
  Bus Selector3/1 -> For Iterator Subsystem/4(outlier_ratio)  "<outlier_ratio>"
  gradient_angle/3(ga_c_out) -> Product4/2
  gradient_angle/4(ga_d_out) -> Product5/2
  gradient_angle/1(ga_a_out) -> Product2/2
  gradient_angle/6(ga_f_out) -> Product7/2
  Bus Selector2/2 -> For Iterator Subsystem/3(sigma)  "<inv_covariance>"
  Product5/1 -> point_gradient/4(ga_d)
  Product3/1 -> point_gradient/2(ga_b)
  set_jacobian/1(jacobian) -> For Iterator Subsystem/8(set_jacobian)
  Bus Selector1/1 -> Product9/1, Product8/1, Product7/1, Product6/1, Product5/1, Product4/1, Product3/1, Product2/1, For Iterator Subsystem/1(data)  "<scan>"
  Bus Selector/1 -> Add/1  "<eig_pose>"
  gradient_angle/7(ga_g_out) -> Product8/2
  Product8/1 -> point_gradient/7(ga_g)
  gradient_angle/8(ga_h_out) -> Product9/2
  Math Function2/1 -> Add4/1
  Product6/1 -> point_gradient/5(ga_e)
  Bus Selector2/1 -> For Iterator Subsystem/2(myu)  "<centroid>"
  localizer_ptr/1 -> Bus Selector3/1
  gradient_angle/5(ga_e_out) -> Product6/2
  gradient_angle/2(ga_b_out) -> Product3/2
  Add/1 -> Product/1
  Bus Selector/3 -> Bus Selector1/1  "<problem>"
  Product7/1 -> point_gradient/6(ga_f)
  Product9/1 -> point_gradient/8(ga_h)
  For Iterator Subsystem/2(jacobian_out) -> Product1/1
  Product/1 -> angle_params/1(pose)  "current_state"
  Add4/1 -> Product1/2, Product/2  "step_direction"
  Product2/1 -> point_gradient/1(ga_a)
  Bus Selector/2 -> Math Function2/1  "<opt_direction>"
  Bus Creator/1 -> initial_objective_function_value/1
  Bus Selector1/2 -> Bus Selector2/1  "<map>"
  point_gradient/1(hessian) -> For Iterator Subsystem/9(set_gradient)
  Bus Selector3/3 -> For Iterator Subsystem/6(voxel_size_y)  "<y>"
  Bus Selector3/4 -> For Iterator Subsystem/7(voxel_size_z)  "<z>"
  phi/1 -> Bus Selector/1
  Bus Selector3/2 -> For Iterator Subsystem/5(voxel_size_x)  "<x>"
  Product4/1 -> point_gradient/3(ga_c)
  step_size/1 -> Bus Creator/1, Add/2  "step_size"
  For Iterator Subsystem/1(score_out) -> Bus Creator/2  "value"
  Product1/1 -> Bus Creator/3  "derivative"

== system NDT_Localization/observation_callback/check_localizer/If Action Subsystem/register_measurement_impl/If Action Subsystem/If Action Subsystem/solve/If Action Subsystem1/For Iterator Subsystem/compute_next_step/If Action Subsystem1/psi_t/objective_function ==
  step_size : Inport
  phi : Inport  Port=2
  localizer_ptr : Inport  Port=3
  Action Port : ActionPort
  Add : Sum
  Add4 : Sum  Inputs=+
  Bus Creator : BusCreator  Inputs=3
  Bus Selector : BusSelector  OutputSignals=eig_pose,opt_direction,problem
  Bus Selector1 : BusSelector  OutputSignals=scan,map
  Bus Selector2 : BusSelector  OutputSignals=vx.centroid,vx.inv_covariance
  Bus Selector3 : BusSelector  OutputSignals=outlier_ratio,localizer_config.map_config.voxel_size.x,localizer_config.map_config.voxel_size.y,localizer_config.map_config.voxel_size.z
  For Iterator Subsystem : Subsystem  TreatAsAtomicUnit=on
  Math Function2 : Math  Operator=square
  Product : Product
  Product{1..9} (9 alike) : Product  Multiplication=Matrix(*)
  angle_params : Subsystem
  gradient_angle : Subsystem
  point_gradient : MATLAB Function  TreatAsAtomicUnit=on
  set_jacobian : MATLAB Function  TreatAsAtomicUnit=on
  objective_function_value : Outport
  wires:
  Add/1 -> Product/1
  step_size/1 -> Bus Creator/1, Add/2  "step_size"
  Product/1 -> angle_params/1(pose)  "current_state"
  Bus Selector/1 -> Add/1  "<eig_pose>"
  Add4/1 -> Product1/2, Product/2  "step_direction"
  phi/1 -> Bus Selector/1
  Bus Selector/2 -> Math Function2/1  "<opt_direction>"
  Math Function2/1 -> Add4/1
  Bus Selector/3 -> Bus Selector1/1  "<problem>"
  For Iterator Subsystem/2(jacobian_out) -> Product1/1
  Product1/1 -> Bus Creator/3  "derivative"
  Product9/1 -> point_gradient/8(ga_h)
  Product8/1 -> point_gradient/7(ga_g)
  Bus Selector2/2 -> For Iterator Subsystem/3(sigma)  "<inv_covariance>"
  gradient_angle/4(ga_d_out) -> Product5/2
  Product7/1 -> point_gradient/6(ga_f)
  Product6/1 -> point_gradient/5(ga_e)
  gradient_angle/6(ga_f_out) -> Product7/2
  Bus Selector1/1 -> Product9/1, Product8/1, Product7/1, Product6/1, Product5/1, Product4/1, Product3/1, Product2/1, For Iterator Subsystem/1(data)  "<scan>"
  point_gradient/1(hessian) -> For Iterator Subsystem/9(set_gradient)
  gradient_angle/2(ga_b_out) -> Product3/2
  gradient_angle/3(ga_c_out) -> Product4/2
  gradient_angle/7(ga_g_out) -> Product8/2
  gradient_angle/5(ga_e_out) -> Product6/2
  gradient_angle/8(ga_h_out) -> Product9/2
  Product5/1 -> point_gradient/4(ga_d)
  Product3/1 -> point_gradient/2(ga_b)
  Product4/1 -> point_gradient/3(ga_c)
  angle_params/1(params) -> gradient_angle/1(params)
  set_jacobian/1(jacobian) -> For Iterator Subsystem/8(set_jacobian)
  Bus Selector1/2 -> Bus Selector2/1  "<map>"
  gradient_angle/1(ga_a_out) -> Product2/2
  Product2/1 -> point_gradient/1(ga_a)
  Bus Selector2/1 -> For Iterator Subsystem/2(myu)  "<centroid>"
  localizer_ptr/1 -> Bus Selector3/1
  Bus Selector3/1 -> For Iterator Subsystem/4(outlier_ratio)  "<outlier_ratio>"
  Bus Selector3/2 -> For Iterator Subsystem/5(voxel_size_x)  "<x>"
  Bus Selector3/3 -> For Iterator Subsystem/6(voxel_size_y)  "<y>"
  Bus Selector3/4 -> For Iterator Subsystem/7(voxel_size_z)  "<z>"
  For Iterator Subsystem/1(score_out) -> Bus Creator/2  "value"
  Bus Creator/1 -> objective_function_value/1

== system NDT_Localization/observation_callback/check_localizer/If Action Subsystem/register_measurement_impl/If Action Subsystem/If Action Subsystem/solve/If Action Subsystem1/For Iterator Subsystem/compute_next_step/If Action Subsystem1/For Iterator Subsystem/If Action Subsystem/If Action Subsystem ==
  psi_t : Inport
  f_l : Inport  Port=2
  f_u : Inport  Port=3
  Action Port : ActionPort  ActionPortLabel=if(u1 > 0)
  a_t : Outport

== system NDT_Localization/observation_callback/check_localizer/If Action Subsystem/register_measurement_impl/If Action Subsystem/If Action Subsystem/solve/If Action Subsystem1/For Iterator Subsystem/compute_next_step/If Action Subsystem1/For Iterator Subsystem/If Action Subsystem/If Action Subsystem1 ==
  phi_t : Inport
  f_l : Inport  Port=2
  f_u : Inport  Port=3
  Action Port : ActionPort  ActionPortLabel=else
  a_t : Outport

== system NDT_Localization/observation_callback/check_localizer/If Action Subsystem/register_measurement_impl/If Action Subsystem/If Action Subsystem/solve/If Action Subsystem1/For Iterator Subsystem/compute_next_step/If Action Subsystem1/For Iterator Subsystem/If Action Subsystem/If Action Subsystem2 ==
  Action Port : ActionPort  ActionPortLabel=if(u1 > 0)
  a_t : Constant  Value=0.0
  a_t_out : Outport
  wires:
  a_t/1 -> a_t_out/1

== system NDT_Localization/observation_callback/check_localizer/If Action Subsystem/register_measurement_impl/If Action Subsystem/If Action Subsystem/solve/If Action Subsystem1/For Iterator Subsystem/compute_next_step/If Action Subsystem1/For Iterator Subsystem/If Action Subsystem/If Action Subsystem3 ==
  a_t : Inport
  localizer_ptr : Inport  Port=2
  aux_function : Inport  Port=3
  phi : Inport  Port=4
  psi : Inport  Port=5
  Action Port : ActionPort  ActionPortLabel=else
  Bus Selector : BusSelector  OutputSignals=value,derivative
  Constant : Constant  Value=0.0
  Data Type Conversion : DataTypeConversion  OutDataTypeStr=uint8  SaturateOnIntegerOverflow=off  RndMeth=Floor
  Data Type Conversion1 : DataTypeConversion  OutDataTypeStr=uint8  SaturateOnIntegerOverflow=off  RndMeth=Floor
  If : If  IfExpression=u1 ~= 0
  If Action Subsystem : Subsystem  TreatAsAtomicUnit=on
  If Action Subsystem1 : Subsystem  TreatAsAtomicUnit=on
  If Action Subsystem2 : Subsystem  TreatAsAtomicUnit=on
  If Action Subsystem3 : Subsystem  TreatAsAtomicUnit=on
  If2 : If  IfExpression=u1 ~= 0
  Logical Operator : Logic  AllPortsSameDT=off  OutDataTypeStr=boolean
  Logical Operator1 : Logic  AllPortsSameDT=off  OutDataTypeStr=boolean
  Merge : Merge
  Relational Operator : RelationalOperator  Operator=<=  OutDataTypeStr=boolean  RndMeth=Simplest  InputSameDT=off
  Relational Operator1 : RelationalOperator  Operator=>  OutDataTypeStr=boolean  RndMeth=Simplest  InputSameDT=off
  phi_t : Subsystem  TreatAsAtomicUnit=on
  psi_t : Subsystem
  Out1 : Outport
  wires:
  psi/1 -> If Action Subsystem2/2(psi), psi_t/2(psi)  "psi"
  a_t/1 -> phi_t/1(a_t), psi_t/1(a_t)  "a_t"
  phi/1 -> If Action Subsystem3/2(phi), If Action Subsystem/1(phi), phi_t/2(phi)  "phi"
  localizer_ptr/1 -> If Action Subsystem/2(localizer_ptr), psi_t/3(localizer_ptr), phi_t/3(localizer_ptr)
  psi_t/1(psi_t) -> If Action Subsystem2/1(psi_t), Bus Selector/1
  Bus Selector/1 -> Relational Operator/1  "<value>"
  Bus Selector/2 -> Relational Operator1/1  "<derivative>"
  Data Type Conversion/1 -> If2/1
  If2/1 -> If Action Subsystem/Action
  Constant/1 -> Relational Operator/2, Relational Operator1/2
  Relational Operator1/1 -> Logical Operator/2
  Relational Operator/1 -> Logical Operator/1
  Logical Operator/1 -> Logical Operator1/2
  aux_function/1 -> If Action Subsystem1/1(aux_function), Logical Operator1/1
  Logical Operator1/1 -> Data Type Conversion/1
  If2/2 -> If Action Subsystem1/Action
  If Action Subsystem/3(aux_function_out) -> Merge/1
  If Action Subsystem1/1(aux_function_out) -> Merge/2
  Merge/1 -> Data Type Conversion1/1
  Data Type Conversion1/1 -> If/1
  If/1 -> If Action Subsystem2/Action
  If/2 -> If Action Subsystem3/Action
  If Action Subsystem/1(f_l_out) -> If Action Subsystem3/3(f_l), If Action Subsystem2/3(f_l)
  If Action Subsystem/2(f_u_out) -> If Action Subsystem3/4(f_u), If Action Subsystem2/4(f_u)
  phi_t/1(phi_t) -> If Action Subsystem3/1(phi_t)

== system NDT_Localization/observation_callback/check_localizer/If Action Subsystem/register_measurement_impl/If Action Subsystem/If Action Subsystem/solve/If Action Subsystem1/For Iterator Subsystem/compute_next_step/If Action Subsystem1/f_l/initial_objective_function/For Iterator Subsystem ==
  data : Inport
  myu : Inport  Port=2
  sigma : Inport  Port=3
  outlier_ratio : Inport  Port=4
  voxel_size_x : Inport  Port=5
  voxel_size_y : Inport  Port=6
  voxel_size_z : Inport  Port=7
  set_jacobian : Inport  Port=8
  set_gradient : Inport  Port=9
  Affine : MATLAB Function  TreatAsAtomicUnit=on
  Delay : Delay  DelayLength=1
  For Iterator : ForIterator  IterationSource=external
  MATLAB Function : MATLAB Function  TreatAsAtomicUnit=on
  Width : Width
  gradient_jaco : Subsystem
  make_c_param : Subsystem
  make_d_param : Subsystem
  score : Subsystem
  score_out : Outport
  jacobian_out : Outport  Port=2
  wires:
  make_c_param/1(c1) -> make_d_param/1(c1)
  voxel_size_z/1 -> make_c_param/4(voxel_size_z)
  outlier_ratio/1 -> make_c_param/1(outlier_ratio)
  make_d_param/2(d2) -> gradient_jaco/9(d2), score/6(d2)
  voxel_size_y/1 -> make_c_param/3(voxel_size_y)
  make_c_param/2(c2) -> make_d_param/2(c2)
  voxel_size_x/1 -> make_c_param/2(voxel_size_x)
  make_d_param/1(d1) -> score/5(d1), gradient_jaco/8(d1)
  Width/1 -> For Iterator/1
  For Iterator/1 -> gradient_jaco/3(index), MATLAB Function/2(index)
  MATLAB Function/1(pt) -> Affine/1(u)
  Affine/1(out) -> score/4(x), gradient_jaco/4(data)
  sigma/1 -> score/2(sigma), gradient_jaco/5(sigma)
  myu/1 -> gradient_jaco/6(myu), score/3(myu)
  score/1(p) -> score_out/1, Delay/1
  Delay/1 -> score/1(score)
  set_jacobian/1 -> gradient_jaco/1(set_jacobian)
  gradient_jaco/1(Out1) -> jacobian_out/1
  set_gradient/1 -> gradient_jaco/2(set_gradient)
  data/1 -> gradient_jaco/7(x), MATLAB Function/1(data), Width/1

== system NDT_Localization/observation_callback/check_localizer/If Action Subsystem/register_measurement_impl/If Action Subsystem/If Action Subsystem/solve/If Action Subsystem1/For Iterator Subsystem/compute_next_step/If Action Subsystem1/f_l/initial_objective_function/angle_params ==
  pose : Inport
  Bus Creator : BusCreator  Inputs=6
  If : If  NumInputs=2  IfExpression=u1 > u2
  If Action Subsystem : Subsystem  TreatAsAtomicUnit=on
  If Action Subsystem1 : Subsystem  TreatAsAtomicUnit=on
  If Action Subsystem2 : Subsystem  TreatAsAtomicUnit=on
  If Action Subsystem3 : Subsystem  TreatAsAtomicUnit=on
  If Action Subsystem4 : Subsystem  TreatAsAtomicUnit=on
  If Action Subsystem5 : Subsystem  TreatAsAtomicUnit=on
  If1 : If  NumInputs=2  IfExpression=u1 > u2
  If2 : If  NumInputs=2  IfExpression=u1 > u2
  MATLAB Function : MATLAB Function  TreatAsAtomicUnit=on
  Merge{,1..5} (6 alike) : Merge
  approx_thresh : Constant  Value=0.00010
  params : Outport
  wires:
  pose/1 -> MATLAB Function/1(u)
  MATLAB Function/1(x) -> If/2, If Action Subsystem1/1(x)
  MATLAB Function/3(z) -> If2/2, If Action Subsystem5/1(z)
  MATLAB Function/2(y) -> If Action Subsystem3/1(y), If1/2
  If Action Subsystem1/1(Out1) -> Merge/2
  If Action Subsystem1/2(Out2) -> Merge1/2
  If Action Subsystem3/1(Out1) -> Merge2/2
  If Action Subsystem3/2(Out2) -> Merge3/2
  If Action Subsystem5/1(Out1) -> Merge4/2
  If Action Subsystem5/2(Out2) -> Merge5/2
  approx_thresh/1 -> If2/1, If1/1, If/1
  If/1 -> If Action Subsystem/Action
  If/2 -> If Action Subsystem1/Action
  If1/1 -> If Action Subsystem2/Action
  If1/2 -> If Action Subsystem3/Action
  If2/2 -> If Action Subsystem5/Action
  If2/1 -> If Action Subsystem4/Action
  If Action Subsystem/1(Out1) -> Merge/1
  If Action Subsystem/2(Out2) -> Merge1/1
  If Action Subsystem2/1(Out1) -> Merge2/1
  If Action Subsystem2/2(Out2) -> Merge3/1
  If Action Subsystem4/1(Out1) -> Merge4/1
  If Action Subsystem4/2(Out2) -> Merge5/1
  Bus Creator/1 -> params/1
  Merge/1 -> Bus Creator/1  "cx"
  Merge1/1 -> Bus Creator/2  "sx"
  Merge2/1 -> Bus Creator/3  "cy"
  Merge3/1 -> Bus Creator/4  "sy"
  Merge4/1 -> Bus Creator/5  "cz"
  Merge5/1 -> Bus Creator/6  "sz"
